simulink model "aem668_project1_simulink"  (R2021b)
settings: Solver=VariableStepAuto  StartTime=0.0  StopTime=15  RelTol=1e-3
values from neighbouring files (symbols this model uses):
  A_lat = [y_b/trim.airspeed, y_p/trim.airspeed, y_r/trim.airspeed - 1, trim.gravity/trim.airspeed*cos(trim.flight_path) ... (first row only)    [p1_668.m]
  B_lat = [0, y_dr/trim.airspeed ... (first row only)    [p1_668.m]
  C_lat = [0 0 1 0 ... (first row only)    [p1_668.m]
undefined symbols (not defined in the file or in its folder): trim
libraries: cstblocks x5, slpidlib x1
settings Model: Creator=Benjamin Lucke  LastModifiedBy=Benjamin Lucke

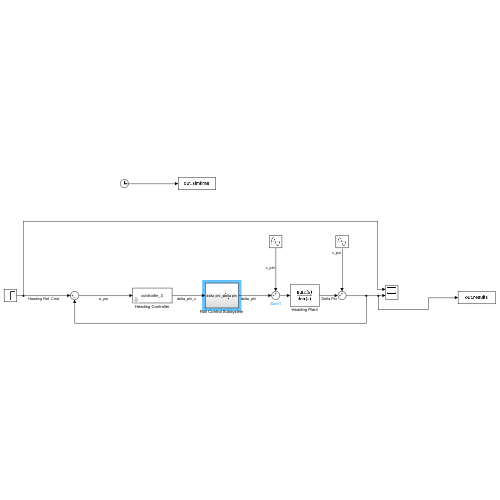
[thumbnail: Simulink's stored preview of the top-level diagram]
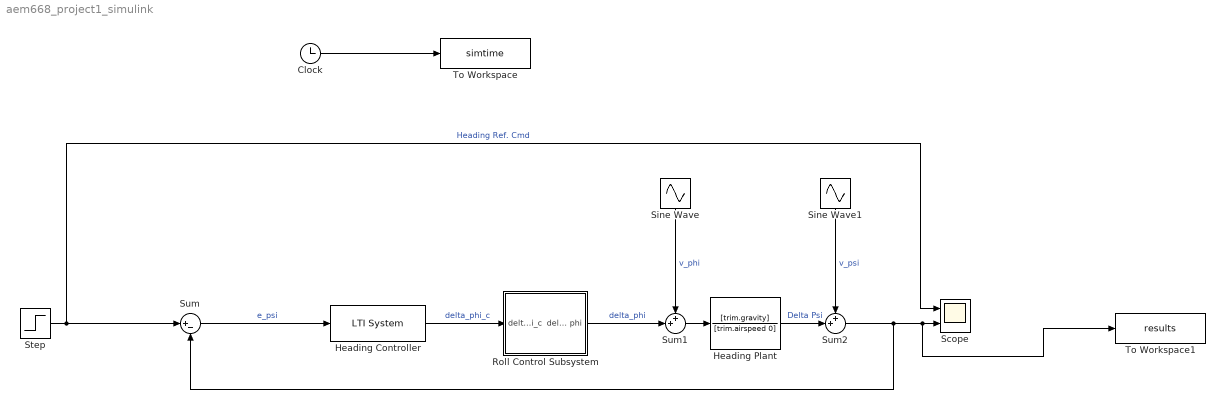
== system aem668_project1_simulink ==
  Clock : Clock
  Heading Controller : cstblocks/LTI System  sys=controller_3  IC=[]
  Heading Plant : TransferFcn  Numerator=[trim.gravity]  Denominator=[trim.airspeed 0]
  Roll Control Subsystem : Subsystem
  Scope : Scope  NumInputPorts=2
  Sine Wave : Sin  Amplitude=.02  Frequency=100  SampleTime=0
  Sine Wave1 : Sin  Amplitude=.02  Frequency=100  SampleTime=0
  Step : Step  After=5  SampleTime=0
  Sum : Sum  Inputs=|+-
  Sum1 : Sum  Inputs=++|
  Sum2 : Sum  Inputs=++|
  To Workspace : ToWorkspace  VariableName=simtime  SaveFormat=Timeseries  SampleTime=-1
  To Workspace1 : ToWorkspace  VariableName=results  SaveFormat=Timeseries  SampleTime=-1
  wires:
  Step/1 -> Scope/1, Sum/1  "Heading Ref. Cmd"
  Heading Controller/1 -> Roll Control Subsystem/1(delta phi_c)  "delta_phi_c"
  Sum/1 -> Heading Controller/1  "e_psi"
  Sine Wave/1 -> Sum1/1  "v_phi"
  Roll Control Subsystem/1(delta phi) -> Sum1/2  "delta_phi"
  Sum1/1 -> Heading Plant/1
  Heading Plant/1 -> Sum2/2  "Delta Psi"
  Sum2/1 -> To Workspace1/1, Scope/2, Sum/2
  Sine Wave1/1 -> Sum2/1  "v_psi"
  Clock/1 -> To Workspace/1

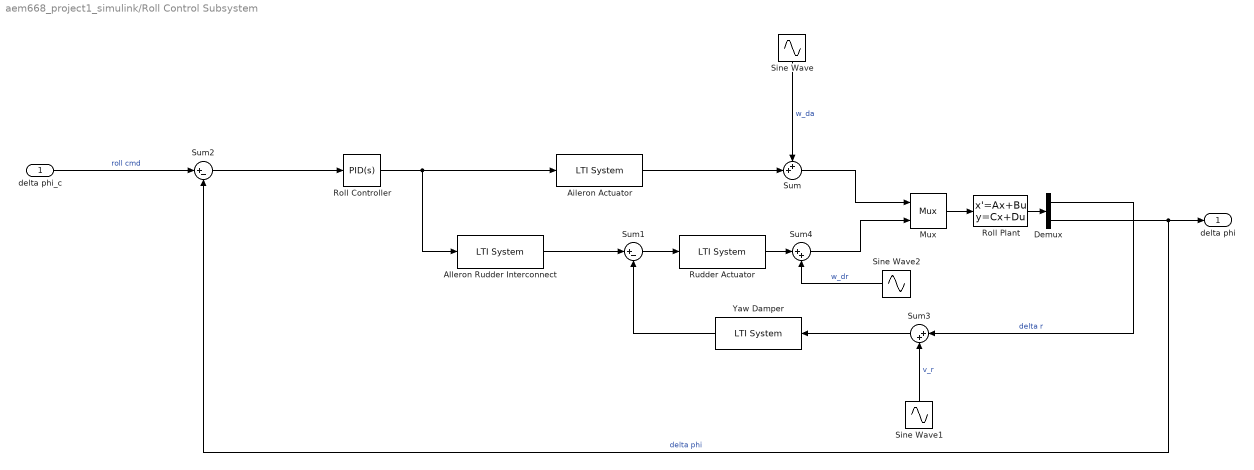
== system aem668_project1_simulink/Roll Control Subsystem ==
  delta phi_c : Inport
  AIleron Rudder Interconnect : cstblocks/LTI System  sys=K_ari  IC=[]
  Aileron Actuator : cstblocks/LTI System  sys=A_a  IC=[]
  Demux : Demux  Outputs=2
  Mux : Mux  Inputs=2
      settings: DisplayOption=signals
  Roll Controller : slpidlib/PID Controller  Controller=PID  Form=Parallel  TimeDomain=Continuous-time  UseExternalTs=off  SampleTime=-1  IntegratorMethod=Forward Euler  FilterMethod=Forward Euler  ControllerParametersSource=internal  P=4.103e04  I=3572e04  D=1962  UseFilter=on  N=100  TunerSelectOption=Transfer Function Based (PID Tuner App)  InitialConditionSource=internal  InitialConditionForIntegrator=0  InitialConditionForFilter=0  DifferentiatorICPrevScaledInput=0  ExternalReset=none  TrackingMode=off  Kt=1  LimitOutput=off  SatLimitsSource=internal  UpperSaturationLimit=inf  LowerSaturationLimit=-inf  LinearizeAsGain=on  AntiWindupMode=none  Kb=1  POutMin=[]  POutMax=[]  IOutMin=[]  IOutMax=[]  DOutMin=[]  DOutMax=[]  NOutMin=[]  NOutMax=[]  SumOutMin=[]  SumOutMax=[]  SaturationOutMin=[]  SaturationOutMax=[]  PParamMin=[]  PParamMax=[]  IParamMin=[]  IParamMax=[]  DParamMin=[]  DParamMax=[]  NParamMin=[]  NParamMax=[]  KbParamMin=[]  KbParamMax=[]  KtParamMin=[]  KtParamMax=[]  KbOutMin=[]  KbOutMax=[]  KtOutMin=[]  KtOutMax=[]  IntegratorOutMin=[]  IntegratorOutMax=[]  FilterOutMin=[]  FilterOutMax=[]  SumI1OutMin=[]  SumI1OutMax=[]  SumI2OutMin=[]  SumI2OutMax=[]  SumI3OutMin=[]  SumI3OutMax=[]  SumI4OutMin=[]  SumI4OutMax=[]  SumDOutMin=[]  SumDOutMax=[]  DifferentiatorOutMin=[]  DifferentiatorOutMax=[]  FilterDiffOutCoefMin=[]  FilterDiffOutCoefMax=[]  ReciprocalOutMin=[]  ReciprocalOutMax=[]  SumDenOutMin=[]  SumDenOutMax=[]  SumNumOutMin=[]  SumNumOutMax=[]  DivideOutMin=[]  DivideOutMax=[]  UdiffTsProdOutMin=[]  UdiffTsProdOutMax=[]  NTsProdOutMin=[]  NTsProdOutMax=[]  UintegralTsProdOutMin=[]  UintegralTsProdOutMax=[]  UngainTsProdOutMin=[]  UngainTsProdOutMax=[]  IntegratorContinuousStateAttributes=''  IntegratorStateMustResolveToSignalObject=off  IntegratorRTWStateStorageClass=Auto  FilterContinuousStateAttributes=''  FilterStateMustResolveToSignalObject=off  FilterRTWStateStorageClass=Auto  ParallelPVariant=InternalParameters  IdealPVariant=Disabled  IVariant=InternalParameters  DVariant=InternalParameters  IntegratorVariant=Continuous  SatVariant=Disabled  AWVariant=Passthrough  PCopyVariant=Disabled  TRVariant=Disabled  FdbkBlocksVariant=Forward  IdealPFdbkVariant=Disabled  SatFdbkVariant=Disabled  DerivativeFilterVariant=ContFilter  NVariant=InternalParameters  NCopyVariant=Disabled  FilterICVariant=InternalICsFilter  IntegratorICVariant=InternalICs  ExternalResetVariant=Disabled  TRSumVariant=Passthrough  SumFdbkVariant=Disabled  SumVariant=Sum_PID  TsampFilterVariant=InternalTs  TsampNgainVariant=Passthrough  TsampIntegralVariant=Passthrough  ExternalSaturationOutDataTypeStr=Inherit: Same as second input
  Roll Plant : StateSpace  A=A_lat  B=B_lat  C=C_lat  D=[0 0; 0 0]  InitialCondition=0
  Rudder Actuator : cstblocks/LTI System  sys=A_r  IC=[]
  Sine Wave : Sin  Amplitude=.01  SampleTime=0
  Sine Wave1 : Sin  Amplitude=.05  Frequency=100  SampleTime=0
  Sine Wave2 : Sin  Amplitude=.01  SampleTime=0
  Sum : Sum  Inputs=++|
  Sum1 : Sum  Inputs=|+-
  Sum2 : Sum  Inputs=|+-
  Sum3 : Sum  Inputs=|++
  Sum4 : Sum  Inputs=|++
  Yaw Damper : cstblocks/LTI System  sys=K_r  IC=[]
  delta phi : Outport
  wires:
  Roll Controller/1 -> Aileron Actuator/1, AIleron Rudder Interconnect/1
  delta phi_c/1 -> Sum2/1  "roll cmd"
  Sum2/1 -> Roll Controller/1
  AIleron Rudder Interconnect/1 -> Sum1/1
  Yaw Damper/1 -> Sum1/2
  Mux/1 -> Roll Plant/1
  Sum1/1 -> Rudder Actuator/1
  Roll Plant/1 -> Demux/1
  Aileron Actuator/1 -> Sum/2
  Sine Wave/1 -> Sum/1  "w_da"
  Sum/1 -> Mux/1
  Sum3/1 -> Yaw Damper/1
  Sine Wave1/1 -> Sum3/2  "v_r"
  Sine Wave2/1 -> Sum4/2  "w_dr"
  Sum4/1 -> Mux/2
  Rudder Actuator/1 -> Sum4/1
  Demux/2 -> Sum2/2, delta phi/1  "delta phi"
  Demux/1 -> Sum3/1  "delta r"
